simulink model "HEV_2_7_26_copy"  (R2026a)
settings: Solver=FixedStepAuto  StopTime=dc_ts{ds_select}.Time(end)
undefined symbols (not defined in the file): C1, C_nom, ds_select, dt, HEV_Param, R1, SOC_init, T_gen_max, V_RC_init
libraries: fl_lib x20, nesl_utility x12, sdl_lib x6, sl_discontinuities x1, simulink_extras x1
settings Model: PacingRate=89  Creator=Aman  LastModifiedBy=Karan Patil
settings SimscapeCC: SimscapeNominalValues="[{\"value\":\"1\",\"unit\":\"A\"},{\"value\":\"1\",\"unit\":\"bar\"},{\"value\":\"1\",\"unit\":\"cm^2\"},{\"value\":\"1\",\"unit\":\"cm^3/s\"},{\"value\":\"1\",\"unit\":\"kJ/kg\"},{\"value\":\"1\",\"unit\":\"kW\"},{\"value\":\"1\",\"unit\":\"l\"},{\"value\":\"1\",\"unit\":\"N\"},{\"value\":\"1\",\"unit\":\"N*m\"},{\"value\":\"1\",\"unit\":\"V\"}]"  SimscapeLogType=none  SimscapeLogDataHistory=5000.0

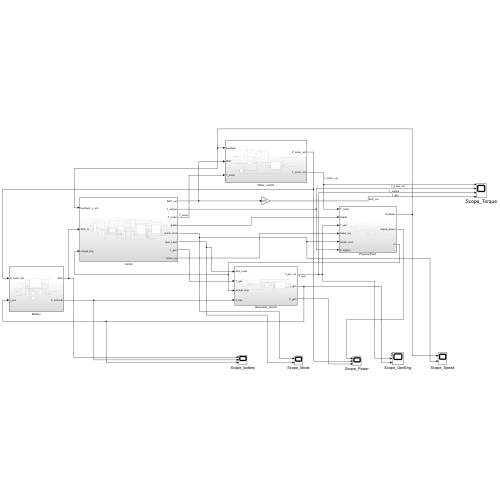
[thumbnail: Simulink's stored preview of the top-level diagram]
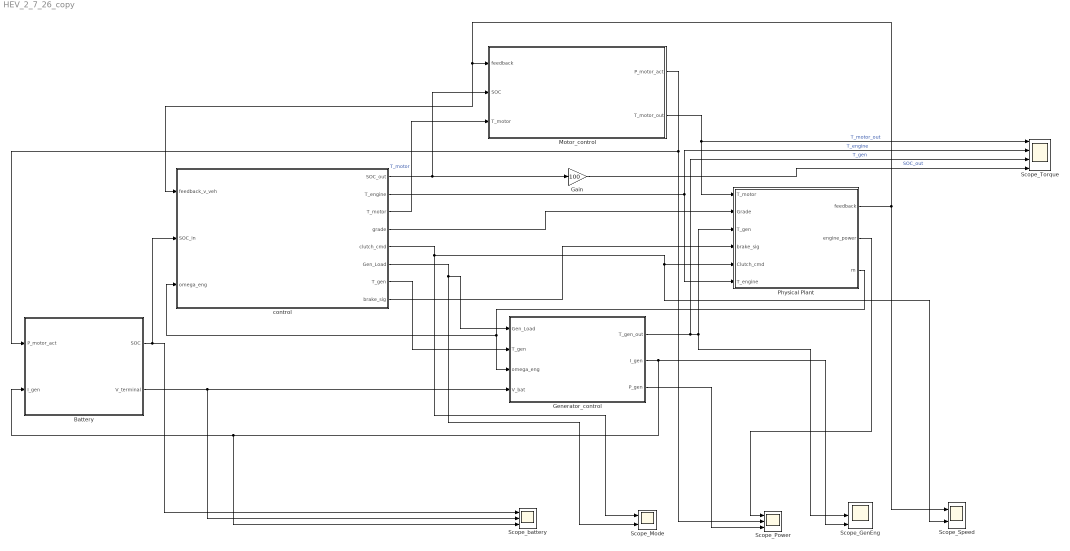
== system HEV_2_7_26_copy ==
  Battery : Subsystem  SystemSampleTime=0.01
  Gain : Gain  Gain=100
  Generator_control : Subsystem
  Motor_control : Subsystem
  Physical Plant : Subsystem
  Scope_GenEng : Scope  NumInputPorts=3
      settings: ActiveDisplayYMinimum=-35.235209426941466  ActiveDisplayYMaximum=313.06846926647512  DataLoggingVariableName=ScopeData6
  Scope_Mode : Scope  NumInputPorts=2
      settings: ActiveDisplayYMinimum=-0.12499999999999997  ActiveDisplayYMaximum=1.125  DataLoggingVariableName=ScopeData5
  Scope_Power : Scope  NumInputPorts=3
      settings: ActiveDisplayYMinimum=-765.7375942803194  ActiveDisplayYMaximum=6218.5415503548766  DataLoggingVariableName=ScopeData4
  Scope_Speed : Scope  NumInputPorts=2
      settings: ActiveDisplayYMinimum=-4.1885981994350328  ActiveDisplayYMaximum=37.4811018776725
  Scope_Torque : Scope  NumInputPorts=4
      settings: ActiveDisplayYMinimum=-11.250026350817844  ActiveDisplayYMaximum=101.25023715736062  DataLoggingVariableName=ScopeData3
  Scope_battery : Scope  NumInputPorts=3
      settings: ActiveDisplayYMinimum=-4.5688448640120694  ActiveDisplayYMaximum=37.733615262780866
  control : Subsystem
  wires:
  control/2(T_engine) -> Scope_Torque/2, Physical Plant/6(T_engine)  "T_engine"
  control/3(T_motor) -> Motor_control/3(T_motor)  "T_motor"
  control/7(T_gen) -> Generator_control/2(T_gen)
  control/4(grade) -> Physical Plant/2(Grade)
  control/5(clutch_cmd) -> Scope_Mode/1, Scope_Speed/2, Physical Plant/5(Clutch_cmd)
  control/6(Gen_Load) -> Scope_Mode/2, Generator_control/1(Gen_Load)
  control/1(SOC_out) -> Motor_control/2(SOC), Gain/1
  Physical Plant/1(feedback) -> control/1(feedback_v_veh), Motor_control/1(feedback), Scope_Speed/1
  Motor_control/1(P_motor_act) -> Scope_Power/2, Battery/1(P_motor_act)
  Battery/1(SOC) -> control/2(SOC_in), Scope_battery/1
  Battery/2(V_terminal) -> Scope_battery/2, Generator_control/4(V_bat)
  Generator_control/1(T_gen_out) -> Scope_Torque/3, Scope_GenEng/2, Physical Plant/3(T_gen)  "T_gen"
  Generator_control/2(I_gen) -> Scope_battery/3, Battery/2(I_gen), Scope_GenEng/3
  Motor_control/2(T_motor_out) -> Physical Plant/1(T_motor), Scope_Torque/1  "T_motor_out"
  Generator_control/3(P_gen) -> Scope_Power/3
  Gain/1 -> Scope_Torque/4  "SOC_out"
  control/8(brake_sig) -> Physical Plant/4(brake_sig)
  Physical Plant/3(m) -> control/3(omega_eng), Generator_control/3(omega_eng)
  Physical Plant/2(engine_power) -> Scope_Power/1

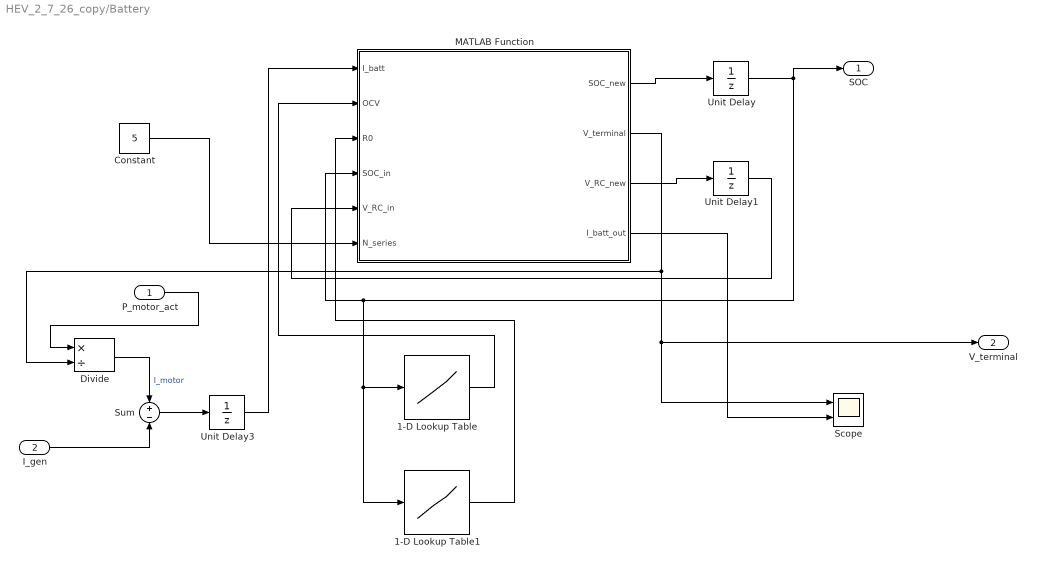
== system HEV_2_7_26_copy/Battery ==
  P_motor_act : Inport
  I_gen : Inport  Port=2
  1-D Lookup Table : Lookup_n-D  NumberOfTableDimensions=1  BreakpointsForDimension1=[0 0.10000000000000001 0.20000000000000001 0.29999999999999999 0.40000000000000002 0.5 0.59999999999999998 0.69999999999999996 0.80000000000000004 0.90000000000000002 1]  Table=[3 3.2000000000000002 3.3500000000000001 3.4500000000000002 3.5499999999999998 3.6499999999999999 3.7200000000000002 3.7799999999999998 3.8500000000000001 3.9300000000000002 4.2000000000000002]  InternalRulePriority=Speed  RndMeth=Simplest
  1-D Lookup Table1 : Lookup_n-D  NumberOfTableDimensions=1  BreakpointsForDimension1=[0;0.20000000000000001;0.5;0.80000000000000004;1]  Table=[0.080000000000000002;0.059999999999999998;0.050000000000000003;0.050000000000000003;0.059999999999999998]  InternalRulePriority=Speed  RndMeth=Simplest
  Constant : Constant  Value=5
  Divide : Product  Inputs=*/
  MATLAB Function : MATLAB Function  TreatAsAtomicUnit=on
  Scope : Scope  NumInputPorts=2
      settings: ActiveDisplayYMinimum=-419.37300934180934  ActiveDisplayYMaximum=3274.3570952541741  DataLoggingVariableName=ScopeData2
  Sum : Sum  Inputs=+-
  Unit Delay : UnitDelay  InitialCondition=SOC_init  SampleTime=-1
  Unit Delay1 : UnitDelay  InitialCondition=V_RC_init  SampleTime=-1
  Unit Delay3 : UnitDelay  SampleTime=0.01
  SOC : Outport
  V_terminal : Outport  Port=2
  wires:
  MATLAB Function/1(SOC_new) -> Unit Delay/1
  Unit Delay/1 -> SOC/1, 1-D Lookup Table1/1, 1-D Lookup Table/1, MATLAB Function/4(SOC_in)
  MATLAB Function/3(V_RC_new) -> Unit Delay1/1
  Unit Delay1/1 -> MATLAB Function/5(V_RC_in)
  MATLAB Function/2(V_terminal) -> Scope/1, V_terminal/1, Divide/2
  P_motor_act/1 -> Divide/1
  Divide/1 -> Sum/1  "I_motor"
  I_gen/1 -> Sum/2
  Sum/1 -> Unit Delay3/1
  MATLAB Function/4(I_batt_out) -> Scope/2
  1-D Lookup Table1/1 -> MATLAB Function/3(R0)
  1-D Lookup Table/1 -> MATLAB Function/2(OCV)
  Unit Delay3/1 -> MATLAB Function/1(I_batt)
  Constant/1 -> MATLAB Function/6(N_series)

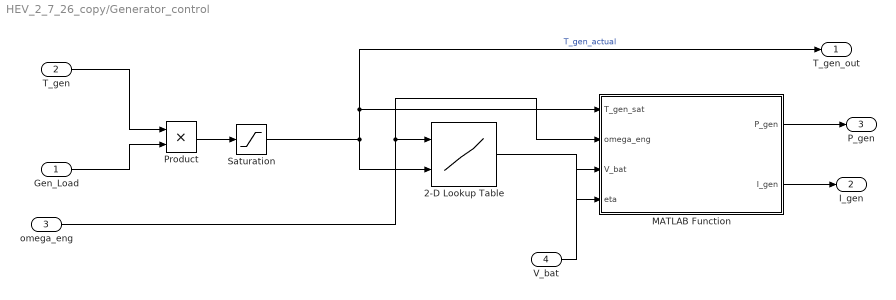
== system HEV_2_7_26_copy/Generator_control ==
  Gen_Load : Inport
  T_gen : Inport  Port=2
  omega_eng : Inport  Port=3
  V_bat : Inport  Port=4
  2-D Lookup Table : Lookup_n-D  BreakpointsForDimension1=[0;50;100;150;200;250;300]  BreakpointsForDimension2=[0;20;40;60;80]  Table=[0.6 0.65 0.7 0.72 0.7;0.68 0.75 0.8 0.82 0.8;0.72 0.82 0.88 0.9 0.89;0.73 0.84 0.9 0.92 0.91;0.72 0.83 0.89 0.91 0.9;0.7 0.8 0.86 0.88 0.87;0.66 0.76 0.82 0.84 0.83]  InternalRulePriority=Speed  RndMeth=Simplest
      settings: InputPortMap=u0,u1
  MATLAB Function : MATLAB Function  TreatAsAtomicUnit=on
  Product : Product
  Saturation : Saturate  UpperLimit=T_gen_max  LowerLimit=0
  T_gen_out : Outport
  I_gen : Outport  Port=2
  P_gen : Outport  Port=3
  wires:
  Product/1 -> Saturation/1
  Saturation/1 -> T_gen_out/1, MATLAB Function/1(T_gen_sat), 2-D Lookup Table/2  "T_gen_actual"
  T_gen/1 -> Product/1
  Gen_Load/1 -> Product/2
  omega_eng/1 -> MATLAB Function/2(omega_eng), 2-D Lookup Table/1
  MATLAB Function/1(P_gen) -> P_gen/1
  2-D Lookup Table/1 -> MATLAB Function/4(eta)
  V_bat/1 -> MATLAB Function/3(V_bat)
  MATLAB Function/2(I_gen) -> I_gen/1

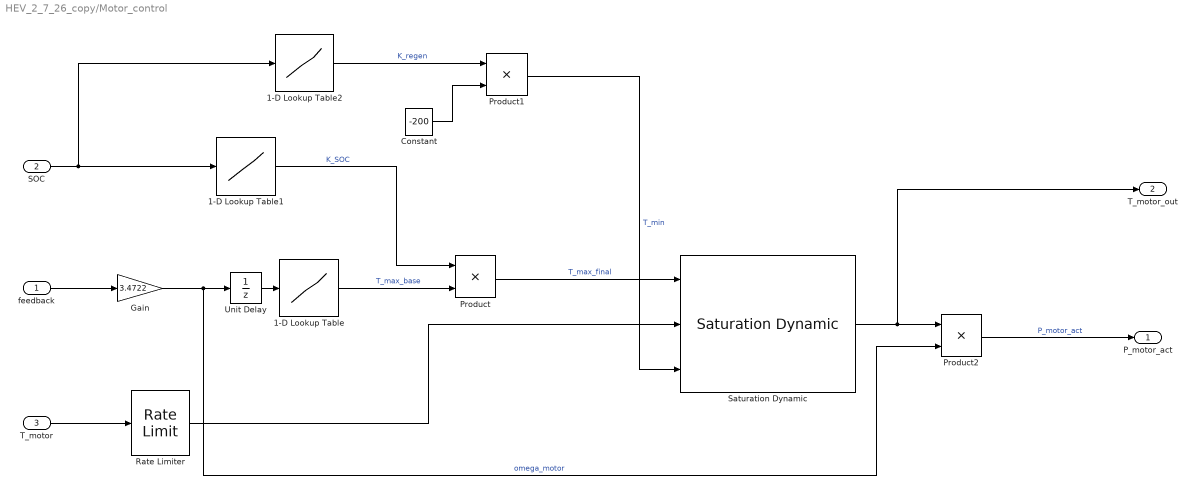
== system HEV_2_7_26_copy/Motor_control ==
  feedback : Inport
  SOC : Inport  Port=2
  T_motor : Inport  Port=3
  1-D Lookup Table : Lookup_n-D  NumberOfTableDimensions=1  BreakpointsForDimension1=[0;50;100;200;400]  Table=[250;250;200;150;100]  InternalRulePriority=Speed  RndMeth=Simplest
  1-D Lookup Table1 : Lookup_n-D  NumberOfTableDimensions=1  BreakpointsForDimension1=[0;0.10000000000000001;0.20000000000000001;1]  Table=[0;0;1;1]  InternalRulePriority=Speed  RndMeth=Simplest
  1-D Lookup Table2 : Lookup_n-D  NumberOfTableDimensions=1  BreakpointsForDimension1=[0;0.80000000000000004;0.84999999999999998;1]  Table=[1;1;0;0]  InternalRulePriority=Speed  RndMeth=Simplest
  Constant : Constant  Value=-200
  Gain : Gain  Gain=3.4722
  Product : Product
  Product1 : Product
  Product2 : Product
  "Rate Limiter " : RateLimiter  RisingSlewLimit=500  FallingSlewLimit=-500  SampleTimeMode=inherited
  Saturation Dynamic : sl_discontinuities/Saturation Dynamic  OutMin=[]  OutMax=[]  OutDataTypeStr=Inherit: Same as second input  OutDataType=fixdt(1, 16)  OutScaling=2^-10  DoSatur=off
      settings: LibrarySourceBlock=|
      | simulink/Discontinuities/Saturation
      | Dynamic
  Unit Delay : UnitDelay  SampleTime=-1
  P_motor_act : Outport
  T_motor_out : Outport  Port=2
  wires:
  feedback/1 -> Gain/1
  Gain/1 -> Unit Delay/1, Product2/2  "omega_motor"
  1-D Lookup Table/1 -> Product/2  "T_max_base"
  SOC/1 -> 1-D Lookup Table2/1, 1-D Lookup Table1/1
  1-D Lookup Table1/1 -> Product/1  "K_SOC"
  Product/1 -> Saturation Dynamic/1  "T_max_final"
  1-D Lookup Table2/1 -> Product1/1  "K_regen"
  Constant/1 -> Product1/2
  Product1/1 -> Saturation Dynamic/3  "T_min"
  T_motor/1 -> "Rate Limiter "/1
  "Rate Limiter "/1 -> Saturation Dynamic/2
  Saturation Dynamic/1 -> Product2/1, T_motor_out/1
  Product2/1 -> P_motor_act/1  "P_motor_act"
  Unit Delay/1 -> 1-D Lookup Table/1

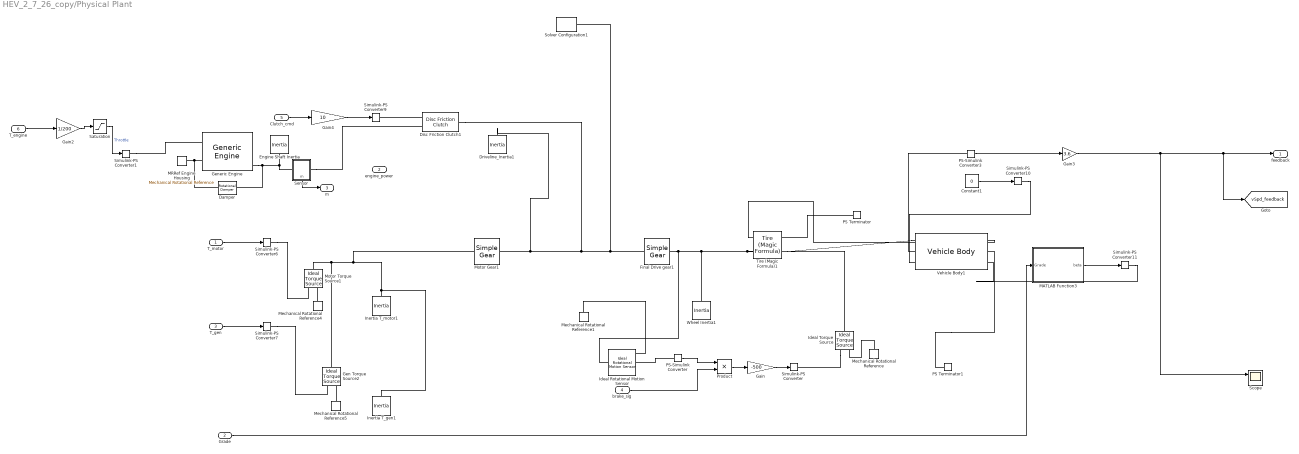
== system HEV_2_7_26_copy/Physical Plant ==
  T_motor : Inport
  Grade : Inport  Port=2
  T_gen : Inport  Port=3
  brake_sig : Inport  Port=4
  Clutch_cmd : Inport  Port=5
  T_engine : Inport  Port=6
  Constant1 : Constant  Value=0
  Damper : fl_lib/Mechanical/Rotational Elements/Rotational Damper  D=HEV_Param.ICE.Friction N*m/(rad/s)  w_specify=off  w_priority=High  w=0 rad/s  w_nominal_specify=off  w_nominal_value=1  w_nominal_unit=rad/s  t_specify=off  t_priority=High  t=0 N*m  t_nominal_specify=off  t_nominal_value=1  t_nominal_unit=N*m
  Disc Friction Clutch1 : sdl_lib/Clutches/Disc Friction Clutch  geometry_model=sdl.enum.friction_geometry.radius  r_eff=130 mm  d_o=150 mm  d_i=100 mm  nS=4  piston_area=0.001 m^2  unidirectional=sdl.enum.directionality.bidirectional  friction_model=sdl.enum.friction_model_TLU_thermal.fixed  mu_w_vector=[0, 100, 1000] rad/s  temperature_TLU=[280, 300, 320] K  mu_static=0.35  mu_static_vector=[.4, .38, .36]  mu_coulomb=0.3  mu_coulomb_vector=[.3, .22, .19]  mu_coulomb_temp_vector=[.3, .28, .25]  mu_coulomb_matrix=[.34, .32, .3; .3, .28, .25; .25, .2, .15]  mu_interp_method=simscape.enum.interpolation.linear  mu_extrap_method=simscape.enum.extrapolation.linear  d_f=1  w_tol=0.001 rad/s  pressure_min=100 Pa  mu_visc=0 N*m*s/rad  initial_state_locked=sdl.enum.initial_lock.unlocked  thermal_mass=50 kJ/K  T_init=300 K
  Driveline_Inertia1 : fl_lib/Mechanical/Rotational Elements/Inertia  inertia=0.01 kg*m^2  num_ports=foundation.enum.numPorts2.one  w_specify=off  w_priority=High  w=0 rad/s  w_nominal_specify=off  w_nominal_value=1  w_nominal_unit=rad/s  t_specify=off  t_priority=None  t=0 N*m  t_nominal_specify=off  t_nominal_value=1  t_nominal_unit=N*m
  Engine Shaft Inertia : fl_lib/Mechanical/Rotational Elements/Inertia  inertia=HEV_Param.ICE.Shaft_Inertia kg*m^2  num_ports=foundation.enum.numPorts2.one  w_specify=on  w_priority=High  w=HEV_Param.Control.Engine_Start_RPM rpm  w_nominal_specify=off  w_nominal_value=1  w_nominal_unit=rad/s  t_specify=off  t_priority=High  t=0 N*m  t_nominal_specify=off  t_nominal_value=1  t_nominal_unit=N*m
  Final Drive gear1 : sdl_lib/Gears/Simple Gear  ratio=2  rotation_direction=sdl.enum.shaftOutputDirection.opposite  friction_model=sdl.enum.gear_efficiencies_load.off  T_noload=0.1 N*m  T_nom=5 N*m  efficiency_nom=0.8  efficiency=0.8  temperature_TLU=[280, 300, 320] K  load_TLU=[1, 5, 10] N*m  efficiency_TLU=[.95, .9, .85]  efficiency_TLU2=[.85, .8, .75; .95, .9, .85; .85, .8, .7]  w_thr=0.01 rad/s  pwr_thr=0.001 W  enable_backlash=false  hardstop_model=simscape.enum.hardstop.smooth  backlash_distance=1e-3 mm  r_base=0.1 m  transition=1e-4 mm  backlash_stiffness=1e6 N/m  backlash_damping=1e3 N*s/m  coeff_rest=0.7  v_tol=0.001 m/s  f_tol=0.001 N  tau=0.1 s  mu_visc=[0, 0] N*m*s/rad  thermal_mass=50 J/K  temperature_specify=off  temperature_priority=High  temperature=300 K  temperature_nominal_specify=off  temperature_nominal_value=1  temperature_nominal_unit=K  x_backlash_specify=off  x_backlash_priority=None  x_backlash=0 mm  x_backlash_nominal_specify=off  x_backlash_nominal_value=1  x_backlash_nominal_unit=mm  f_hardstop_specify=off  f_hardstop_priority=None  f_hardstop=0 N  f_hardstop_nominal_specify=off  f_hardstop_nominal_value=1  f_hardstop_nominal_unit=N  v_backlash_specify=off  v_backlash_priority=None  v_backlash=0 m/s  v_backlash_nominal_specify=off  v_backlash_nominal_value=1  v_backlash_nominal_unit=m/s
  Gain : Gain  Gain=-500
  Gain2 : Gain  Gain=1/200
  Gain3 : Gain  Gain=3.6
  Gain4 : Gain  Gain=10
  Gen Torque Source2 : fl_lib/Mechanical/Mechanical Sources/Ideal Torque Source
  Generic Engine : sdl_lib/Engines & Motors/Generic Engine  input_type=sdl.enum.GenericEngineInputType.NormalizedThrottle  model_parameterization=1  engine_type=1  Trq_max=380 N*m  w_Trq_max=4300 rpm  P_max=HEV_Param.ICE.Max_Power W  w_P_max=HEV_Param.ICE.Speed_At_Max_Power rpm  w_max=HEV_Param.ICE.Max_Speed rpm  w_min=500 rpm  w_tab=[ 500 1000 2e+3 3e+3 4e+3 5e+3 6e+3 7e+3 ] rpm  trq_tab=[ 380 380 380 380 350 280 200 80 ] N*m  pwr_tab=[ 2e+4 4e+4 7.8e+4 1.2e+5 1.45e+5 1.48e+5 1.25e+5 6e+4 ] W  interp_method=1  w_thr=100 rpm  model_inertia=0  inertia=1 kg*m^2  initial_velocity=800 rpm  model_time_constant=0  time_constant=0.2 s  initial_normalized_throttle=0  fc_model=1  fc_per_rev=25 mg/rev  fc_w_tab=[ 1000 2e+3 3e+3 4e+3 5e+3 6e+3 ] rpm  fc_trq_tab=[ 0 80 160 200 240 320 360 400 ] N*m  fc_tab=[ 0.5 0.9 1.4 1.6 1.9 2.7 3.4 4.4; 1 1.7 2.7 3.1 3.6 5 6 7.4; 1.4 2.7 4 4.8 5.6 7.5 8.5 10.5; 2 3.6 5.8 6.7 8 10.4 11.7 13.3; 2.5 4.8 7.9 9.4 10.8 14 16.2 18.6; 3.1 6 10.3 11.9 13.8 18.4 22 26.5 ] g/s  bmep_tab=[ 0 250 500 625 750 1000 1.15e+3 1.25e+3 ] kPa  bsfc_tab=[ 410 380 300 280 270 290 320 380; 410 370 290 270 260 270 285 320; 415 380 290 275 265 270 270 300; 420 390 310 290 285 280 280 285; 430 410 340 320 310 300 310 320; 450 430 370 340 330 330 350 380 ] g/hr/kW  fc_interp_method=1  displaced_volume=400 cm^3  rev_per_cycle=2  idle_speed=0  idle_speed_reference=1000 rpm  tau_controller=1 s  idle_w_thr=1 rpm  redline=0  redline_speed=5000 rpm  tau_redline=1 s  redline_w_thr=1 rpm
  Ideal Rotational Motion Sensor : fl_lib/Mechanical/Mechanical Sensors/Ideal Rotational Motion Sensor  reference=foundation.enum.MeasurementReference.difference  acceleration_port=false  velocity_port=true  position_port=true  wrap_angle=false  offset=0 rad
  Ideal Torque Source : fl_lib/Mechanical/Mechanical Sources/Ideal Torque Source
  Inertia T_gen1 : fl_lib/Mechanical/Rotational Elements/Inertia  inertia=0.01 kg*m^2  num_ports=foundation.enum.numPorts2.one  w_specify=off  w_priority=High  w=0 rad/s  w_nominal_specify=off  w_nominal_value=1  w_nominal_unit=rad/s  t_specify=off  t_priority=None  t=0 N*m  t_nominal_specify=off  t_nominal_value=1  t_nominal_unit=N*m
  Inertia T_motor1 : fl_lib/Mechanical/Rotational Elements/Inertia  inertia=0.01 kg*m^2  num_ports=foundation.enum.numPorts2.one  w_specify=off  w_priority=High  w=0 rad/s  w_nominal_specify=off  w_nominal_value=1  w_nominal_unit=rad/s  t_specify=off  t_priority=None  t=0 N*m  t_nominal_specify=off  t_nominal_value=1  t_nominal_unit=N*m
  MATLAB Function3 : MATLAB Function  TreatAsAtomicUnit=on
  MRRef Engine Housing : fl_lib/Mechanical/Rotational Elements/Mechanical Rotational Reference
  Mechanical Rotational Reference{,1,4..5} (4 alike) : fl_lib/Mechanical/Rotational Elements/Mechanical Rotational Reference
  Motor Gear1 : sdl_lib/Gears/Simple Gear  ratio=2  rotation_direction=sdl.enum.shaftOutputDirection.opposite  friction_model=sdl.enum.gear_efficiencies_load.off  T_noload=0.1 N*m  T_nom=5 N*m  efficiency_nom=0.8  efficiency=0.8  temperature_TLU=[280, 300, 320] K  load_TLU=[1, 5, 10] N*m  efficiency_TLU=[.95, .9, .85]  efficiency_TLU2=[.85, .8, .75; .95, .9, .85; .85, .8, .7]  w_thr=0.01 rad/s  pwr_thr=0.001 W  enable_backlash=false  hardstop_model=simscape.enum.hardstop.smooth  backlash_distance=1e-3 mm  r_base=0.1 m  transition=1e-4 mm  backlash_stiffness=1e6 N/m  backlash_damping=1e3 N*s/m  coeff_rest=0.7  v_tol=0.001 m/s  f_tol=0.001 N  tau=0.1 s  mu_visc=[0, 0] N*m*s/rad  thermal_mass=50 J/K  temperature_specify=off  temperature_priority=High  temperature=300 K  temperature_nominal_specify=off  temperature_nominal_value=1  temperature_nominal_unit=K  x_backlash_specify=off  x_backlash_priority=None  x_backlash=0 mm  x_backlash_nominal_specify=off  x_backlash_nominal_value=1  x_backlash_nominal_unit=mm  f_hardstop_specify=off  f_hardstop_priority=None  f_hardstop=0 N  f_hardstop_nominal_specify=off  f_hardstop_nominal_value=1  f_hardstop_nominal_unit=N  v_backlash_specify=off  v_backlash_priority=None  v_backlash=0 m/s  v_backlash_nominal_specify=off  v_backlash_nominal_value=1  v_backlash_nominal_unit=m/s
  Motor Torque Source1 : fl_lib/Mechanical/Mechanical Sources/Ideal Torque Source
  PS Terminator : fl_lib/Physical Signals/Sinks/PS Terminator
  PS Terminator1 : fl_lib/Physical Signals/Sinks/PS Terminator
  PS-Simulink Converter : nesl_utility/PS-Simulink Converter  PhysicalDomain=network_engine_domain  SubClassName=ps_output  LeftPortType=input  RightPortType=output  PseudoPeriodic=off  Frequencies=[]  VectorFormat=inherit  Unit=inherit  AffineConversion=off
  PS-Simulink Converter3 : nesl_utility/PS-Simulink Converter  PhysicalDomain=network_engine_domain  SubClassName=ps_output  LeftPortType=input  RightPortType=output  PseudoPeriodic=off  Frequencies=[]  VectorFormat=inherit  Unit=m/s  AffineConversion=off
  Product : Product
  Saturation : Saturate  UpperLimit=1  LowerLimit=0
  Scope : Scope  NumInputPorts=2
      settings: ActiveDisplayYMinimum=-253.090340995205  ActiveDisplayYMaximum=376.67362528602291
  Sensor : Subsystem
      settings: PortSchema="{\"entries\":[{\"content\":{\"sides\":[{\"content\":{\"connectorIds\":[\"LConn1\"]},\"type\":\"ConnectorPlacement.EquallySpacedRectSide\",\"uuid\":\"5a33ac70-cd2c-47ff-b866-bd3f3557f685\"},{\"content\":{\"connectorIds\":[\"RConn1\"],\"side\":\"RIGHT\"},\"type\":\"ConnectorPlacement.EquallySpacedRectSide\",\"uuid\":\"5c843a06-af9b-4ac3-9267-bba109437eb6\"},{\"content\":{\"side\":\"TOP\"},\"type\":\"ConnectorPlacement.EquallySpacedRectSide\",\"uuid\":\"fe58ca13-627c-4f53-907b-1080a8c8494c\"},{\"content\":{\"connectorIds\":[\"Out1\"],\"side\":\"BOTTOM\"},\"type\":\"ConnectorPlacement.EquallySpacedRectSide\",\"uuid\":\"ba14817e-a66b-4663-ba7e-b24568ac9611\"}]},\"type\":\"ConnectorPlacement.EquallySpacedConnector\",\"uuid\":\"5d87e06c-df1a-4ca2-879b-92f90cce612e\"}],\"packageUris\":[\"http://schema.mathworks.com/mf0/Connector/R2020b\"],\"version\":\"1.0\"}"
      mask Display: disp('S');
  Simulink-PS Converter : nesl_utility/Simulink-PS Converter  PhysicalDomain=network_engine_domain  SubClassName=ps_input  LeftPortType=input  RightPortType=output  PseudoPeriodic=off  Frequencies=[]  NoiseDistribution=none  NoiseParameters=[]  Unit=1  AffineConversion=off  FilteringAndDerivatives=filter  SimscapeFilterOrder=1  InputFilterTimeConstant=0.01  UdotUserProvided=0
  Simulink-PS Converter1 : nesl_utility/Simulink-PS Converter  PhysicalDomain=network_engine_domain  SubClassName=ps_input  LeftPortType=input  RightPortType=output  PseudoPeriodic=off  Frequencies=[]  NoiseDistribution=none  NoiseParameters=[]  Unit=1  AffineConversion=off  FilteringAndDerivatives=zero  SimscapeFilterOrder=1  InputFilterTimeConstant=0.005  UdotUserProvided=0
  Simulink-PS Converter10 : nesl_utility/Simulink-PS Converter  PhysicalDomain=network_engine_domain  SubClassName=ps_input  LeftPortType=input  RightPortType=output  PseudoPeriodic=off  Frequencies=[]  NoiseDistribution=none  NoiseParameters=[]  Unit=1  AffineConversion=off  FilteringAndDerivatives=provide  SimscapeFilterOrder=1  InputFilterTimeConstant=0.001  UdotUserProvided=0
  Simulink-PS Converter11 : nesl_utility/Simulink-PS Converter  PhysicalDomain=network_engine_domain  SubClassName=ps_input  LeftPortType=input  RightPortType=output  PseudoPeriodic=off  Frequencies=[]  NoiseDistribution=none  NoiseParameters=[]  Unit=rad  AffineConversion=off  FilteringAndDerivatives=provide  SimscapeFilterOrder=1  InputFilterTimeConstant=0.001  UdotUserProvided=0
  Simulink-PS Converter6 : nesl_utility/Simulink-PS Converter  PhysicalDomain=network_engine_domain  SubClassName=ps_input  LeftPortType=input  RightPortType=output  PseudoPeriodic=off  Frequencies=[]  NoiseDistribution=none  NoiseParameters=[]  Unit=N*m  AffineConversion=off  FilteringAndDerivatives=filter  SimscapeFilterOrder=1  InputFilterTimeConstant=0.001  UdotUserProvided=0
  Simulink-PS Converter7 : nesl_utility/Simulink-PS Converter  PhysicalDomain=network_engine_domain  SubClassName=ps_input  LeftPortType=input  RightPortType=output  PseudoPeriodic=off  Frequencies=[]  NoiseDistribution=none  NoiseParameters=[]  Unit=N*m  AffineConversion=off  FilteringAndDerivatives=filter  SimscapeFilterOrder=1  InputFilterTimeConstant=0.001  UdotUserProvided=0
  Simulink-PS Converter9 : nesl_utility/Simulink-PS Converter  PhysicalDomain=network_engine_domain  SubClassName=ps_input  LeftPortType=input  RightPortType=output  PseudoPeriodic=off  Frequencies=[]  NoiseDistribution=none  NoiseParameters=[]  Unit=bar  AffineConversion=off  FilteringAndDerivatives=provide  SimscapeFilterOrder=1  InputFilterTimeConstant=0.001  UdotUserProvided=0
  Solver Configuration1 : nesl_utility/Solver Configuration  PhysicalDomain=network_engine_domain  SubClassName=solver  LeftPortType=input  RightPortType=generic  Tones=[]  Harmonics=[]  SimulateNoise=off  Profile=off  UseLocalSampling=off  EnableSwitchedLinearOptims=on  FrequencyDomain=off  UseCCode=off  RelTol=0.001  AbsTol=0.001  MinStep=1e-09  ToWorkspace=off  RevertToSquareIcSolve=off  NumHomotopyIterations=100  PhasorMode=off  PhasorModeNumHarmonics=1  ConsistencySolver=NEWTON_XTOL_AFTER_FTOL  CanonicalOrdering=UNORDERED  OptimizeIntermediates=UNOPTIMIZED  IndexReductionMethod=DerivativeReplacement  DoDC=off  ResidualTolerance=1e-09  ConsistencyTolSource=GLOBAL  ConsistencyAbsTol=0.001  ConsistencyRelTol=0.001  ConsistencyTolFactor=0.001  UseLocalSolver=off  LocalSolverChoice=NE_BACKWARD_EULER_ADVANCER  ResolveIndetEquations=on  FunctionEvalNumThread=1  LocalSolverSampleTime=0.001  DoFixedCost=off  MaxNonlinIter=3  MaxModeIter=2  ComputeImpulses=off  ImpulseIterations=2  LinearAlgebra=auto  LinearAlgebraNumThread=0  EquationFormulation=NE_TIME_EF  DelaysMemoryBudget=1024  AutomaticFiltering=on  FilteringTimeConstant=0.001  PartitionStorageMethod=AS_NEEDED  PartitionMemoryBudget=1024  PartitionMethod=ROBUST  MultibodyUseLocalSolver=off  MultibodyLocalSolverChoice=ODE1  MultibodyLocalSolverSampleTime=0.001
  Tire (Magic Formula)1 : sdl_lib/Tires & Vehicles/Tire (Magic Formula)  parameterization=sdl.enum.magic_tire_model.peak  F_z1=3000 N  F_x1=3500 N  kappa1=10  B_m=10  C_m=1.9  D_m=1  E_m=0.97  fz0=4000 N  p_Cx=1.685  p_Dx=[1.21, -.037]  p_Ex=[.344, .095, -.02, 0]  p_Kx=[21.51, -.163, .245]  p_Hx=[-.002, .002]  p_Vx=[0, 0]  rolling_radius_model=sdl.enum.RollingRadiusParameterization.Constant  r_e=0.3 m  r_0=0.3 m  breff=8.39  dreff=0.26  freff=0.074  q_re0=0.99  q_v1=0.008  longvl=17 m/s  cz=5e5 N/m  model_resistance=false  resistance_model=sdl.enum.rollingResistanceParameterization.constant  coeff=0.015  p_tire=250e3 Pa  alpha=-0.003  beta=0.97  coeff_a=84e-4  coeff_b=6.2e-4 s/m  coeff_c=1.6e-4 s^2/m^2  p_tire0=240e3 Pa  fz0_resistance=4000 N  vH0=16 m/s  q_Sy=[.0082, 0, .0014, .001, 0, 0, 1.08, -.5]  v_thr=0.001 m/s  enable_scaling_coefficients=false  lfzO=1  lcx=1  lmux=1  lex=1  lkx=1  lhx=1  lvx=1  lmy=1  model_compliance=sdl.enum.compliance.off  stiffness=1e6 N/m  damping=1000 N*s/m  model_inertia=sdl.enum.model_inertia.off  inertia=1 kg*m^2  initial_velocity=0 rad/s  vxlow=1 m/s  v_tr_thr=0.1 m/s  kpumin=-1.5  kpumax=1.5
  Vehicle Body1 : sdl_lib/Tires & Vehicles/Vehicle Body  mass=1200 kg  n_w=2  x_f=1.4 m  x_r=1.6 m  y_c=0.5 m  mass_var=false  g=9.81 m/s^2  liftoff_warning=false  area=3 m^2  Cd_var=false  Cd=0.4  rho=1.18 kg/m^3  model_pitch=false  inertia=4000 kg*m^2  suspension_model=sdl.enum.linearTLU.linear  k_f=1e4 N/m  b_f=1e4 N*s/m  k_r=1e4 N/m  b_r=1e4 N*s/m  k_f_TLU=[-2000, -1000, 0, 1000, 2000] N  x_f_TLU=[-.4, -.2, 0, .2, .4] m  b_f_TLU=[-200, -100, 0, 100, 200] N  v_f_TLU=[-4, -2, 0, 2, 4] m/s  k_r_TLU=[-2000, -1000, 0, 1000, 2000] N  x_r_TLU=[-.4, -.2, 0, .2, .4] m  b_r_TLU=[-200, -100, 0, 100, 200] N  v_r_TLU=[-4, -2, 0, 2, 4] m/s  interp_method=simscape.enum.interpolation.linear  extrap_method=simscape.enum.extrapolation.linear  model_hardstop=false  upper_bound_f=.25 m  lower_bound_f=-.25 m  stop_k_f=1e6 N/m  stop_b_f=150 N*s/m  upper_bound_r=.25 m  lower_bound_r=-.25 m  stop_k_r=1e6 N/m  stop_b_r=150 N*s/m  initial_pitch=0 rad  initial_pitch_rate=0 rad/s  v_specify=off  v_priority=High  v=0 m/s  v_nominal_specify=off  v_nominal_value=1  v_nominal_unit=m/s
  Wheel Inertia1 : fl_lib/Mechanical/Rotational Elements/Inertia  inertia=0.01 kg*m^2  num_ports=foundation.enum.numPorts2.one  w_specify=off  w_priority=High  w=0 rad/s  w_nominal_specify=off  w_nominal_value=1  w_nominal_unit=rad/s  t_specify=off  t_priority=None  t=0 N*m  t_nominal_specify=off  t_nominal_value=1  t_nominal_unit=N*m
  feedback : Outport
  engine_power : Outport  Port=2
  m : Outport  Port=3
  tag scope: vSpd_feedback=global
  wires:
  MATLAB Function3/1(beta) -> Simulink-PS Converter11/1
  Grade/1 -> MATLAB Function3/1(Grade)
  PS-Simulink Converter3/1 -> Gain3/1
  Constant1/1 -> Simulink-PS Converter10/1
  T_motor/1 -> Simulink-PS Converter6/1
  T_gen/1 -> Simulink-PS Converter7/1
  PS-Simulink Converter/1 -> Product/1
  brake_sig/1 -> Product/2
  Product/1 -> Gain/1
  Gain/1 -> Simulink-PS Converter/1
  Gain3/1 -> [vSpd_feedback], feedback/1, Scope/1
  Gain2/1 -> Saturation/1
  T_engine/1 -> Gain2/1
  Saturation/1 -> Simulink-PS Converter1/1  "Throttle"
  Clutch_cmd/1 -> Gain4/1
  Gain4/1 -> Simulink-PS Converter9/1
  Sensor/1(m) -> m/1
  connections:
  Motor Torque Source1/LConn1 -- Gen Torque Source2/LConn1 -- Motor Gear1/LConn1 -- Inertia T_motor1/LConn1 -- Inertia T_gen1/LConn1
  Driveline_Inertia1/LConn1 -- Disc Friction Clutch1/RConn1 -- Final Drive gear1/LConn1 -- Solver Configuration1/RConn1 -- Motor Gear1/RConn1
  PS Terminator/LConn1 -- Tire (Magic Formula)1/RConn1
  Simulink-PS Converter6/RConn1 -- Motor Torque Source1/RConn1
  Simulink-PS Converter10/RConn1 -- Vehicle Body1/LConn3
  Simulink-PS Converter11/RConn1 -- Vehicle Body1/RConn3
  Vehicle Body1/LConn2 -- PS-Simulink Converter3/LConn1
  Mechanical Rotational Reference5/LConn1 -- Gen Torque Source2/RConn2
  PS Terminator1/LConn1 -- Vehicle Body1/RConn2
  Tire (Magic Formula)1/RConn2 -- Vehicle Body1/LConn1
  Mechanical Rotational Reference4/LConn1 -- Motor Torque Source1/RConn2
  Simulink-PS Converter7/RConn1 -- Gen Torque Source2/RConn1
  PS-Simulink Converter/LConn1 -- Ideal Rotational Motion Sensor/RConn2
  Mechanical Rotational Reference/LConn1 -- Ideal Torque Source/RConn2
  Final Drive gear1/RConn1 -- Tire (Magic Formula)1/LConn2 -- Ideal Torque Source/LConn1 -- Wheel Inertia1/LConn1 -- Ideal Rotational Motion Sensor/LConn1
  Vehicle Body1/RConn1 -- Tire (Magic Formula)1/LConn1
  Ideal Torque Source/RConn1 -- Simulink-PS Converter/RConn1
  Mechanical Rotational Reference1/LConn1 -- Ideal Rotational Motion Sensor/RConn1
  Disc Friction Clutch1/LConn1 -- Simulink-PS Converter9/RConn1
  Damper/LConn1 -- Engine Shaft Inertia/LConn1 -- Sensor/LConn1 -- Generic Engine/RConn3
  Generic Engine/LConn2 -- MRRef Engine Housing/LConn1 -- Damper/RConn1
  Simulink-PS Converter1/RConn1 -- Generic Engine/LConn1
  Sensor/RConn1 -- Disc Friction Clutch1/LConn2

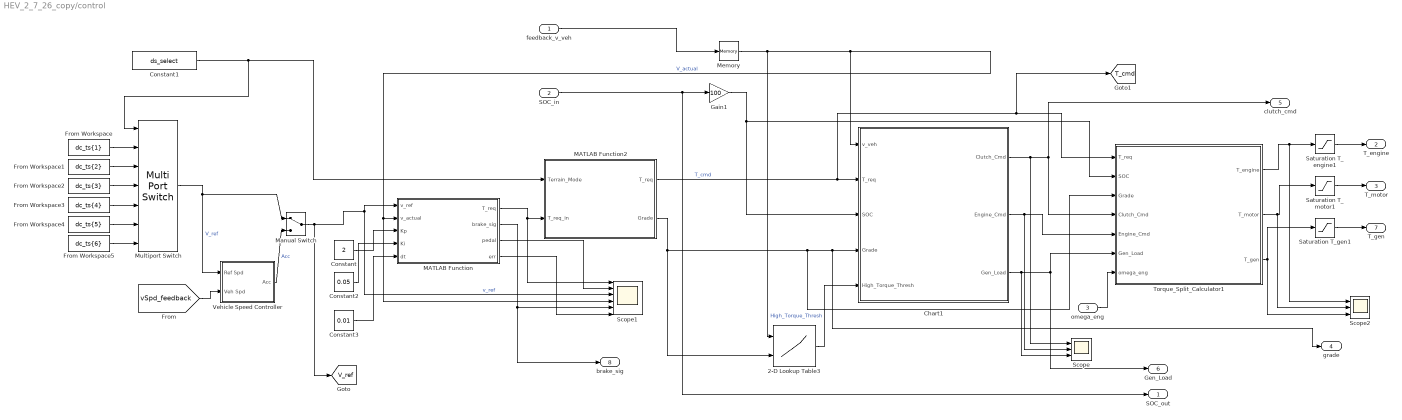
== system HEV_2_7_26_copy/control ==
  feedback_v_veh : Inport
  SOC_in : Inport  Port=2
  omega_eng : Inport  Port=3
  2-D Lookup Table3 : Lookup_n-D  BreakpointsForDimension1=[0;20;40;60;70;80;100;120]  BreakpointsForDimension2=[0 5 10]  Table=[100 80 60;120 100 80;140 120 100;155 135 115;145 125 105;130 110 90;115 95 75;95 80 65]  InternalRulePriority=Speed  RndMeth=Simplest
      settings: InputPortMap=u0,u1
  Chart1 : Stateflow chart  TreatAsAtomicUnit=on
  Constant : Constant  Value=2
  Constant1 : Constant  Value=ds_select
  Constant2 : Constant  Value=0.05
  Constant3 : Constant  Value=0.01
  From Workspace : FromWorkspace  VariableName=dc_ts{1}  OutDataTypeStr=double
  From Workspace1 : FromWorkspace  VariableName=dc_ts{2}  OutDataTypeStr=double
  From Workspace2 : FromWorkspace  VariableName=dc_ts{3}  OutDataTypeStr=double  SampleTime=dt  OutputAfterFinalValue=Holding final value
  From Workspace3 : FromWorkspace  VariableName=dc_ts{4}  OutDataTypeStr=double  SampleTime=dt  OutputAfterFinalValue=Holding final value
  From Workspace4 : FromWorkspace  VariableName=dc_ts{5}  OutDataTypeStr=double  SampleTime=dt  OutputAfterFinalValue=Holding final value
  From Workspace5 : FromWorkspace  VariableName=dc_ts{6}  OutDataTypeStr=double  SampleTime=dt  OutputAfterFinalValue=Holding final value
  Gain1 : Gain  Gain=100
  MATLAB Function : MATLAB Function  TreatAsAtomicUnit=on
  MATLAB Function2 : MATLAB Function  TreatAsAtomicUnit=on
  Manual Switch : ManualSwitch
  Memory : Memory
  Multiport Switch : MultiPortSwitch  Inputs=6  SaturateOnIntegerOverflow=off  InputSameDT=off
  Saturation T_engine1 : Saturate  UpperLimit=450  LowerLimit=-450
  Saturation T_gen1 : Saturate  UpperLimit=200  LowerLimit=0
  Saturation T_motor1 : Saturate  UpperLimit=200  LowerLimit=-80
  Scope : Scope  NumInputPorts=3
      settings: ActiveDisplayYMinimum=-0.60052689778822044  ActiveDisplayYMaximum=1.4077457230092125  DataLoggingVariableName=ScopeData7
  Scope1 : Scope  NumInputPorts=6
      settings: ActiveDisplayYMinimum=-28.678754866925559  ActiveDisplayYMaximum=98.438093266476756  DataLoggingVariableName=ScopeData8
  Scope2 : Scope  NumInputPorts=3
      settings: ActiveDisplayYMinimum=-52.578193571128651  ActiveDisplayYMaximum=219.7865386049842  DataLoggingVariableName=ScopeData9
  Torque_Split_Calculator1 : MATLAB Function  TreatAsAtomicUnit=on
  Vehicle Speed Controller : Subsystem
  SOC_out : Outport
  T_engine : Outport  Port=2
  T_motor : Outport  Port=3
  grade : Outport  Port=4
  clutch_cmd : Outport  Port=5
  Gen_Load : Outport  Port=6
  T_gen : Outport  Port=7
  brake_sig : Outport  Port=8
  tag scope: T_cmd=global, V_ref=global
  wires:
  MATLAB Function2/1(T_req) -> [T_cmd], Torque_Split_Calculator1/1(T_req), Chart1/2(T_req)  "T_cmd"
  MATLAB Function2/2(Grade) -> 2-D Lookup Table3/2, Torque_Split_Calculator1/3(Grade), Chart1/4(Grade), grade/1
  2-D Lookup Table3/1 -> Chart1/5(High_Torque_Thresh)  "High_Torque_Thresh"
  Chart1/1(Clutch_Cmd) -> Scope/1, clutch_cmd/1, Torque_Split_Calculator1/4(Clutch_Cmd)
  Chart1/2(Engine_Cmd) -> Scope/2, Torque_Split_Calculator1/5(Engine_Cmd)
  Chart1/3(Gen_Load) -> Scope/3, Gen_Load/1, Torque_Split_Calculator1/6(Gen_Load)
  Torque_Split_Calculator1/1(T_engine) -> Scope2/1, Saturation T_engine1/1
  Torque_Split_Calculator1/2(T_motor) -> Scope2/2, Saturation T_motor1/1
  Torque_Split_Calculator1/3(T_gen) -> Saturation T_gen1/1, Scope2/3
  Saturation T_engine1/1 -> T_engine/1
  Saturation T_motor1/1 -> T_motor/1
  Saturation T_gen1/1 -> T_gen/1
  Memory/1 -> 2-D Lookup Table3/1, Scope1/4, MATLAB Function/2(v_actual), Chart1/1(v_veh)  "V_actual"
  feedback_v_veh/1 -> Memory/1
  SOC_in/1 -> SOC_out/1, Gain1/1
  From Workspace3/1 -> Multiport Switch/5
  From Workspace5/1 -> Multiport Switch/7
  From Workspace2/1 -> Multiport Switch/4
  Multiport Switch/1 -> Vehicle Speed Controller/1(Ref Spd), Manual Switch/1  "V_ref"
  From Workspace/1 -> Multiport Switch/2
  From Workspace1/1 -> Multiport Switch/3
  From Workspace4/1 -> Multiport Switch/6
  Constant1/1 -> MATLAB Function2/1(Terrain_Mode), Multiport Switch/1
  Constant/1 -> MATLAB Function/3(Kp)
  MATLAB Function/1(T_req) -> Scope1/1, MATLAB Function2/2(T_req_in)
  omega_eng/1 -> Torque_Split_Calculator1/7(omega_eng)
  Gain1/1 -> Chart1/3(SOC), Torque_Split_Calculator1/2(SOC)
  MATLAB Function/3(pedal) -> Scope1/2
  MATLAB Function/2(brake_sig) -> brake_sig/1, Scope1/5
  MATLAB Function/4(err) -> Scope1/6
  [vSpd_feedback] -> Vehicle Speed Controller/2(Veh Spd)
  Vehicle Speed Controller/1(Acc) -> Manual Switch/2  "Acc"
  Manual Switch/1 -> [V_ref], Scope1/3, MATLAB Function/1(v_ref)  "v_ref"
  Constant2/1 -> MATLAB Function/4(Ki)
  Constant3/1 -> MATLAB Function/5(dt)

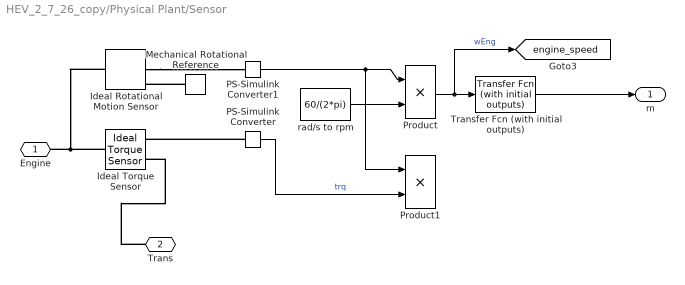
== system HEV_2_7_26_copy/Physical Plant/Sensor ==
  Ideal Rotational Motion Sensor : fl_lib/Mechanical/Mechanical Sensors/Ideal Rotational Motion Sensor  reference=foundation.enum.MeasurementReference.difference  acceleration_port=false  velocity_port=true  position_port=true  wrap_angle=simscape.enum.onoff.off  offset=0 rad
  Ideal Torque Sensor : fl_lib/Mechanical/Mechanical Sensors/Ideal Torque Sensor
  Mechanical Rotational Reference : fl_lib/Mechanical/Rotational Elements/Mechanical Rotational Reference
  PS-Simulink Converter : nesl_utility/PS-Simulink Converter  PhysicalDomain=network_engine_domain  SubClassName=ps_output  LeftPortType=input  RightPortType=output  PseudoPeriodic=off  Frequencies=[]  VectorFormat=1-D array  Unit=N*m  AffineConversion=off
  PS-Simulink Converter1 : nesl_utility/PS-Simulink Converter  PhysicalDomain=network_engine_domain  SubClassName=ps_output  LeftPortType=input  RightPortType=output  PseudoPeriodic=off  Frequencies=[]  VectorFormat=1-D array  Unit=rad/s  AffineConversion=off
  Product : Product  RndMeth=Zero
  Product1 : Product  RndMeth=Zero
  Transfer Fcn (with initial outputs) : simulink_extras/Additional Linear/Transfer Fcn (with initial outputs)  N=[1]  D=[0.01 1]  Y0=HEV_Param.Control.Engine_Start_RPM  U0=HEV_Param.Control.Engine_Start_RPM
  rad/s to rpm : Constant  Value=60/(2*pi)
  Engine : PMIOPort  Side=Left
  Trans : PMIOPort  Port=2  Side=Right
  m : Outport
  tag scope: engine_speed=global
  wires:
  PS-Simulink Converter/1 -> Product1/2  "trq"
  Product/1 -> [engine_speed], Transfer Fcn (with initial outputs)/1  "wEng"
  PS-Simulink Converter1/1 -> Product/1, Product1/1
  rad/s to rpm/1 -> Product/2
  Transfer Fcn (with initial outputs)/1 -> m/1
  connections:
  Ideal Torque Sensor/LConn1 -- Engine/RConn1 -- Ideal Rotational Motion Sensor/LConn1
  Trans/RConn1 -- Ideal Torque Sensor/RConn1
  PS-Simulink Converter/LConn1 -- Ideal Torque Sensor/RConn2
  Ideal Rotational Motion Sensor/RConn2 -- PS-Simulink Converter1/LConn1
  Mechanical Rotational Reference/LConn1 -- Ideal Rotational Motion Sensor/RConn1

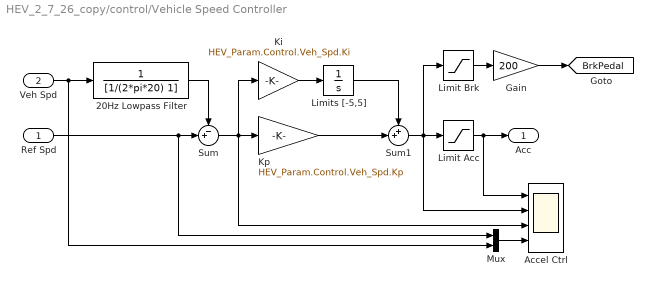
== system HEV_2_7_26_copy/control/Vehicle Speed Controller ==
  Ref Spd : Inport
  Veh Spd : Inport  Port=2
  20Hz Lowpass Filter : TransferFcn  Denominator=[1/(2*pi*20) 1]
  Accel Ctrl : Scope  NumInputPorts=4
      settings: ActiveDisplayYMinimum=-4.21362433267499  ActiveDisplayYMaximum=37.852231165114141  DataLoggingMaxPoints=100  DataLoggingVariableName=ScopeData11
  Gain : Gain  Gain=200
  Ki : Gain  Gain=HEV_Param.Control.Veh_Spd.Ki
  Kp : Gain  Gain=HEV_Param.Control.Veh_Spd.Kp
  Limit Acc : Saturate  UpperLimit=1  LowerLimit=0
  Limit Brk : Saturate  UpperLimit=0  LowerLimit=-inf
  Limits [-5,5] : Integrator  LimitOutput=on  UpperSaturationLimit=5  LowerSaturationLimit=-5
  Mux : Mux  Inputs=2
  Sum : Sum  Inputs=-+|
  Sum1 : Sum  Inputs=++|
  Acc : Outport  VectorParamsAs1DForOutWhenUnconnected=off
  tag scope: BrkPedal=global
  wires:
  Limit Acc/1 -> Acc/1, Accel Ctrl/1
  Veh Spd/1 -> 20Hz Lowpass Filter/1, Mux/2
  Sum1/1 -> Limit Brk/1, Limit Acc/1, Accel Ctrl/2
  Sum/1 -> Ki/1, Kp/1, Accel Ctrl/3
  Ki/1 -> Limits [-5,5]/1
  Kp/1 -> Sum1/2
  Limits [-5,5]/1 -> Sum1/1
  20Hz Lowpass Filter/1 -> Sum/1
  Mux/1 -> Accel Ctrl/4
  Limit Brk/1 -> Gain/1
  Gain/1 -> [BrkPedal]
  Ref Spd/1 -> Sum/2, Mux/1

== matlab function HEV_2_7_26_copy/Battery/MATLAB Function ==
  data: I_batt input; SOC_new output; OCV input; R0 input; SOC_in input; V_RC_in input; V_terminal output; V_RC_new output; I_batt_out output; dt parameter; C_nom parameter; R1 parameter; C1 parameter; N_series input
function [SOC_new, V_terminal, V_RC_new, I_batt_out] = ...
         BatteryECM(I_batt, OCV, R0, SOC_in, V_RC_in, dt, C_nom, R1, C1, N_series)

%% 1. SOC integration (Coulomb counting) — unchanged, this part is correct
dSOC    = -I_batt * dt / (C_nom * 3600);
SOC_new = SOC_in + dSOC;
SOC_new = max(0, min(1, SOC_new));

%% 2. RC pair dynamics — unchanged at cell level, scale at the end
alpha = exp(-dt/(R1*C1));
V_RC_new = alpha*V_RC_in + R1*(1-alpha)*I_batt;

%% 3. Terminal voltage — scale OCV, R0 drop, and V_RC up to pack level
OCV_pack       = OCV * N_series;
R0_pack_drop   = I_batt * R0 * N_series;
V_RC_pack      = V_RC_new * N_series;

V_terminal = OCV_pack - R0_pack_drop - V_RC_pack;
V_terminal = max(2.5*N_series, min(4.3*N_series, V_terminal)); % pack-level clamp

%% 4. Pass-through
I_batt_out = I_batt;
end

== matlab function HEV_2_7_26_copy/Generator_control/MATLAB Function ==
  data: T_gen_sat input; P_gen output; I_gen output; omega_eng input; V_bat input; eta input; I_max_charge parameter
function [P_gen,I_gen] = GeneratorPower(T_gen_sat, omega_eng, V_bat, eta, I_max_charge)

% Electrical power generation
P_gen = T_gen_sat * omega_eng * eta;

% Avoid divide-by-zero
V_nom_min = 1;
V_safe = max(V_bat, V_nom_min);

% Charging current
I_gen = P_gen / V_safe;

% Current limit
I_gen = min(I_gen, I_max_charge);

% No negative charging current
I_gen = max(I_gen,0);

end

== matlab function HEV_2_7_26_copy/control/MATLAB Function ==
  settings: updateMethod=DISCRETE
  data: v_ref input; T_req output; v_actual input; Kp input; brake_sig output; pedal output; err output; Ki input; dt input
function [T_req, brake_sig, pedal, err] = DriverPI(v_ref, v_actual, Kp, Ki, dt)
% 1. Initialize memory
persistent int_err T_req_filt
if isempty(int_err)
    int_err = 0;
    T_req_filt = 0;
end

% 2. Error calculation
err = v_ref - v_actual;

% 3. Proper Time-Based Integration
int_err = int_err + (err * dt);

% 4. Anti-Windup (Clamp the integrator memory safely)
if Ki ~= 0
    int_limit = 1 / abs(Ki);
    int_err = max(-int_limit, min(int_limit, int_err));
end

% 5. PI Control Law
pedal_unsat = (Kp * err) + (Ki * int_err);
pedal = max(-1, min(1, pedal_unsat));

% 6. Torque Calculation
T_req_raw = max(0, pedal) * 280;
brake_sig = max(0, -pedal);

% 7. Low-Pass Filter (Smooths the output)
alpha = 0.02;
T_req_filt = T_req_filt + alpha * (T_req_raw - T_req_filt);
T_req = T_req_filt;
end

== stateflow chart HEV_2_7_26_copy/control/Chart1 ==
  state Vehicle_Active
    state Regen_Braking
      entry: Engine_Cmd = 0; Clutch_Cmd = 0; Gen_Load = 1;
    state Propulsion
      state Series_mode
        entry: Engine_Cmd = 1; Clutch_Cmd = 0; Gen_Load = 1;
      state Parallel_mode
        entry: Engine_Cmd = 1; Clutch_Cmd = 1; Gen_Load = 0;
      state Series_Parallel_mode
        entry: Engine_Cmd = 1; Clutch_Cmd = 1; Gen_Load = 1;
      (default) -> Series_mode
      Series_Parallel_mode -> Series_mode [order 2] : [v_veh < 70 || Grade >= 5]
      Series_mode -> Series_Parallel_mode [order 2] : [v_veh > 80 && SOC < 30]
      Series_mode -> Parallel_mode [order 1] : [v_veh > 80 && SOC > 40 && Grade < 5]
      Parallel_mode -> Series_mode [order 1] : [v_veh < 70 || Grade >= 5]
      Parallel_mode -> Series_Parallel_mode [order 2] : [SOC < 30 || Grade >= 5 && T_req > High_Torque_Thresh]
      Series_Parallel_mode -> Parallel_mode [order 1] : [SOC > 40]
    (default) -> Propulsion
    Propulsion -> Regen_Braking : [T_req < 0]
    Regen_Braking -> Propulsion : [T_req >= 0]
  state Vehicle_Standby
    entry: Engine_Cmd = 0; Clutch_Cmd = 0; Gen_Load = 0;
  (default) -> Vehicle_Standby
  Vehicle_Standby -> Vehicle_Active : [v_veh >= 0.5 || T_req > 0]
  Vehicle_Active -> Vehicle_Standby : [v_veh < 0.5 && T_req == 0]
  data: v_veh input; T_req input; SOC input; Grade input; Clutch_Cmd output; Engine_Cmd output; High_Torque_Thresh input; Gen_Load output

== matlab function HEV_2_7_26_copy/control/MATLAB Function2 ==
  data: Terrain_Mode input; T_req_in input; T_req output; Grade output
function [T_req, Grade] = generate_terrain_scenario(Terrain_Mode, T_req_in)
% #codegen
% This block generates simulated vehicle states based on selected terrain.
%
% Input:
%   Terrain_Mode - 1 = City, 2 = Highway, 3 = Mountain, etc.
%
% Outputs:
%   T_req  - Driver torque request in Nm
%   Grade  - Road gradient in %

    switch Terrain_Mode
        case 1
            % drive cycle 1
            T_req = T_req_in;    % Nm
            Grade = 0.0;         % flat road
        case 2
            % drive cycle 2
            T_req = T_req_in;    % Nm
            Grade = 1.0;         % slight road grade
        case 3
            % drive cycle 3
            T_req = T_req_in;    % Nm
            Grade = 8.0;         % steep uphill road  
        case 4
            % drive cycle 4
            T_req = T_req_in;    % Nm
            Grade = 0.0;         % flat road
        case 5
            % drive cycle 5
            T_req = T_req_in;    % Nm
            Grade = 1.0;         % slight road grade
        case 6
            % drive cycle 6
            T_req = T_req_in;    % Nm
            Grade = 8.0;         % steep uphill road  
        otherwise
            % DEFAULT / FAILSAFE
            T_req = 0.0;         % Safely zero out torque demand
            Grade = 0.0;         % Assume flat ground
    end
end

== matlab function HEV_2_7_26_copy/Physical Plant/MATLAB Function3 ==
  data: Grade input; beta output
function beta = grade_to_angle(Grade)
%#codegen
beta = atan(Grade/100);
end

== matlab function HEV_2_7_26_copy/control/Torque_Split_Calculator1 ==
  data: T_req input; SOC input; T_engine output; Grade input; T_motor output; T_gen output; Clutch_Cmd input; Engine_Cmd input; Gen_Load input; omega_eng input
function [T_engine, T_motor, T_gen] = Torque_Split_Dynamic(...
     T_req, SOC, Grade, Clutch_Cmd, Engine_Cmd, Gen_Load,omega_eng)

%  CONSTANTS & VEHICLE PARAMETERS
g            = 9.81;        % m/s^2 - Gravity
m_veh        = 1200;        % kg    - Vehicle mass
r_wheel      = 0.3;        % m     - Wheel radius

%% POWERTRAIN PARAMETERS
T_engine_max = 200;         % Nm    - Max engine torque
T_motor_max  = 150;         % Nm    - Max motor torque
T_gen_max    = 150;         % Nm    - Max generator torque capacity
T_engine_opt = 120;         % Nm    - Engine best efficiency torque


eta_gen      = 0.90;        % -     - Generator efficiency
eta_motor    = 0.92;        % -     - Motor efficiency
eta_clutch   = 0.97;        % -     - Clutch mechanical efficiency

%% SOC THRESHOLDS
SOC_low      = 30;          % %     - Low battery threshold
SOC_high     = 80;          % %     - High battery threshold
SOC_target   = 60;          % %     - Ideal SOC target
k_soc        = 0.5;         % -     - SOC error gain

%%  PHYSICS CALCULATIONS

theta = atan(Grade / 100);               % [radians]
F_grade = m_veh * g * sin(theta);        % Grade force [N]


W_soc = max(0, min(1, (SOC - SOC_low) / (SOC_high - SOC_low)));
delta_T_charge = k_soc * (SOC_target - SOC); 

%%  COMMAND-BASED TORQUE SPLIT

% Initialize all values
T_engine = 0; T_motor = 0; T_gen = 0;
omega_engine = omega_eng;

if Engine_Cmd == 0 && Clutch_Cmd == 0 && Gen_Load == 1
    % --- STANDBY or REGEN BRAKING ---
    if T_req < 0 
        T_motor = -abs(T_req) * eta_motor;
        T_motor = max(T_motor, -T_motor_max);              
    else
        T_motor  = 0;
    end

elseif Engine_Cmd == 1 && Clutch_Cmd == 0 && Gen_Load == 1
    % --- SERIES MODE ---
    T_motor = min(T_req, T_motor_max);
    
    if SOC >= SOC_high
        T_engine = 0;
    else
        T_engine = T_engine_opt + delta_T_charge;
        T_engine = max(0, min(T_engine, T_engine_max));
    end
    
    T_gen = T_engine; % Generator absorbs mechanical torque directly

elseif Engine_Cmd == 1 && Clutch_Cmd == 1 && Gen_Load == 0
    % --- PARALLEL MODE ---
    T_grade_motor = F_grade * r_wheel;                  
    
    T_engine = (1 - W_soc) * T_engine_max;
    T_engine = min(T_engine, T_req);
    
    T_motor  = (T_req - (T_engine * eta_clutch)) + T_grade_motor;
    T_motor  = max(0, min(T_motor, T_motor_max));
    T_gen    = 0;

elseif Engine_Cmd == 1 && Clutch_Cmd == 1 && Gen_Load == 1
    % --- SERIES-PARALLEL MODE ---
    T_engine = T_engine_opt;
    
    if T_engine >= T_req
        % Engine has surplus. Calculate torque gap and route to generator.
        T_surplus = T_engine - T_req;
        T_gen     = T_surplus;
        T_motor   = 0;
    else
        % Engine has deficit. Motor must assist.
        T_motor = min(T_req - T_engine, T_motor_max);
        T_gen   = 0;
    end
end


T_engine = max(0, min(T_engine, T_engine_max));
T_motor  = max(-T_motor_max, min(T_motor, T_motor_max));

% BUG 4 FIXED: Clamped to T_gen_max instead of T_engine_max
T_gen    = max(0, min(T_gen, T_gen_max)); 

end
